simulink model "FailureModesGen"  (R2018b)
settings: configuration reference "Physics" (kept outside this file)
model workspace (MAT data in the model file):
  m = 1000
values from neighbouring files (symbols this model uses):
  P_SimDetectFailures = 1    [FailureModesGen.sldd]
  P_SimFailureBrakeMode = 0.0    [FailureModesGen.sldd]
  P_SimFailureBrakeStepEndTime_s = 200.0    [FailureModesGen.sldd]
  P_SimFailureBrakeStepTime_s = -1.0    [FailureModesGen.sldd]
  P_SimFailureIMU1Mode = 0.0    [FailureModesGen.sldd]
  P_SimFailureIMU1StepEndTime_s = 200.0    [FailureModesGen.sldd]
  P_SimFailureIMU1StepTime_s = -1.0    [FailureModesGen.sldd]
  P_SimFailureIMU2Mode = 0.0    [FailureModesGen.sldd]
  P_SimFailureIMU2StepEndTime_s = 200.0    [FailureModesGen.sldd]
  P_SimFailureIMU2StepTime_s = -1.0    [FailureModesGen.sldd]
  P_SimFailureLoc1Mode = 0.0    [FailureModesGen.sldd]
  P_SimFailureLoc1StepEndTime_s = 200.0    [FailureModesGen.sldd]
  P_SimFailureLoc1StepTime_s = -1.0    [FailureModesGen.sldd]
  P_SimFailureLoc2Mode = 0.0    [FailureModesGen.sldd]
  P_SimFailureLoc2StepEndTime_s = 200.0    [FailureModesGen.sldd]
  P_SimFailureLoc2StepTime_s = -1.0    [FailureModesGen.sldd]
  P_SimFailureModeDetectionDelay = 6.0    [FailureModesGen.sldd]
  P_SimFailureSteeringActuatorMode = 0.0    [FailureModesGen.sldd]
  P_SimFailureSteeringActuatorStepEndTime_s = 200.0    [FailureModesGen.sldd]
  P_SimFailureSteeringActuatorStepTime_s = -1.0    [FailureModesGen.sldd]
  P_SimFailureSteeringMode = 0.0    [FailureModesGen.sldd]
  P_SimFailureSteeringStepEndTime_s = 200.0    [FailureModesGen.sldd]
  P_SimFailureSteeringStepTime_s = -1.0    [FailureModesGen.sldd]
  P_SimFailureTorqueMode = 0.0    [FailureModesGen.sldd]
  P_SimFailureTorqueStepEndTime_s = 200.0    [FailureModesGen.sldd]
  P_SimFailureTorqueStepTime_s = -1.0    [FailureModesGen.sldd]
  P_SimFailureVehicleMode = 0.0    [FailureModesGen.sldd]
  P_SimFailureVehicleStepEndTime_s = 200.0    [FailureModesGen.sldd]
  P_SimFailureVehicleStepTime_s = -1.0    [FailureModesGen.sldd]
  P_SimFailureVel1Mode = 0.0    [FailureModesGen.sldd]
  P_SimFailureVel1StepEndTime_s = 200.0    [FailureModesGen.sldd]
  P_SimFailureVel1StepTime_s = -1.0    [FailureModesGen.sldd]
  P_SimFailureVel2Mode = 0.0    [FailureModesGen.sldd]
  P_SimFailureVel2StepEndTime_s = 200.0    [FailureModesGen.sldd]
  P_SimFailureVel2StepTime_s = -1.0    [FailureModesGen.sldd]
  P_SimFailureWheelspeedsMode = 0.0    [FailureModesGen.sldd]
  P_SimFailureWheelspeedsStepEndTime_s = 200.0    [FailureModesGen.sldd]
  P_SimFailureWheelspeedsStepTime_s = -1.0    [FailureModesGen.sldd]
settings Model: DataDictionary=FailureModesGen.sldd  PauseTimes=9.280  Creator=wischnewski  LastModifiedBy=ge34qer

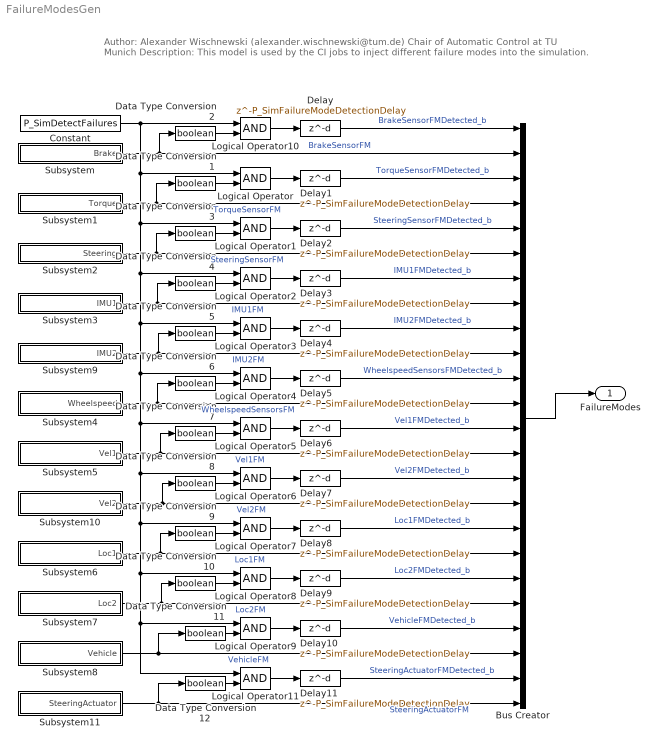
== system FailureModesGen ==
  note: Author: Alexander Wischnewski (alexander.wischnewski@tum.de)
      | Chair of Automatic Control at TU Munich
      |
      | Description: This model is used by the CI jobs to inject different failure modes into the simulation.
  Bus Creator : BusCreator  Inputs=24
  Constant : Constant  Value=P_SimDetectFailures
  Data Type Conversion{1..12} (12 alike) : DataTypeConversion  OutDataTypeStr=boolean
  Delay{,1..11} (12 alike) : Delay  DelayLength=P_SimFailureModeDetectionDelay  InitialCondition=0
  Logical Operator{,1..11} (12 alike) : Logic  AllPortsSameDT=off  OutDataTypeStr=boolean
  Subsystem : Subsystem
  Subsystem1 : Subsystem
  Subsystem10 : Subsystem
  Subsystem11 : Subsystem
  Subsystem2 : Subsystem
  Subsystem3 : Subsystem
  Subsystem4 : Subsystem
  Subsystem5 : Subsystem
  Subsystem6 : Subsystem
  Subsystem7 : Subsystem
  Subsystem8 : Subsystem
  Subsystem9 : Subsystem
  FailureModes : Outport  OutDataTypeStr=Bus: FailureModes
  wires:
  Logical Operator10/1 -> Delay/1
  Delay/1 -> Bus Creator/1  "BrakeSensorFMDetected_b"
  Subsystem/1(Brake) -> Data Type Conversion2/1, Bus Creator/2  "BrakeSensorFM"
  Subsystem1/1(Torque) -> Data Type Conversion1/1, Bus Creator/4  "TorqueSensorFM"
  Delay1/1 -> Bus Creator/3  "TorqueSensorFMDetected_b"
  Subsystem2/1(Steering) -> Data Type Conversion3/1, Bus Creator/6  "SteeringSensorFM"
  Logical Operator1/1 -> Delay2/1
  Delay2/1 -> Bus Creator/5  "SteeringSensorFMDetected_b"
  Delay3/1 -> Bus Creator/7  "IMU1FMDetected_b"
  Subsystem3/1(IMU1) -> Data Type Conversion4/1, Bus Creator/8  "IMU1FM"
  Logical Operator3/1 -> Delay4/1
  Delay4/1 -> Bus Creator/9  "IMU2FMDetected_b"
  Subsystem9/1(IMU2) -> Data Type Conversion5/1, Bus Creator/10  "IMU2FM"
  Logical Operator4/1 -> Delay5/1
  Subsystem4/1(Wheelspeed) -> Data Type Conversion6/1, Bus Creator/12  "WheelspeedSensorsFM"
  Delay5/1 -> Bus Creator/11  "WheelspeedSensorsFMDetected_b"
  Logical Operator5/1 -> Delay6/1
  Delay6/1 -> Bus Creator/13  "Vel1FMDetected_b"
  Subsystem5/1(Vel1) -> Data Type Conversion7/1, Bus Creator/14  "Vel1FM"
  Logical Operator6/1 -> Delay7/1
  Delay7/1 -> Bus Creator/15  "Vel2FMDetected_b"
  Subsystem10/1(Vel2) -> Data Type Conversion8/1, Bus Creator/16  "Vel2FM"
  Logical Operator7/1 -> Delay8/1
  Delay8/1 -> Bus Creator/17  "Loc1FMDetected_b"
  Subsystem6/1(Loc1) -> Data Type Conversion9/1, Bus Creator/18  "Loc1FM"
  Logical Operator8/1 -> Delay9/1
  Delay9/1 -> Bus Creator/19  "Loc2FMDetected_b"
  Subsystem7/1(Loc2) -> Data Type Conversion10/1, Bus Creator/20  "Loc2FM"
  Logical Operator9/1 -> Delay10/1
  Delay10/1 -> Bus Creator/21  "VehicleFMDetected_b"
  Subsystem8/1(Vehicle) -> Data Type Conversion11/1, Bus Creator/22  "VehicleFM"
  Bus Creator/1 -> FailureModes/1
  Constant/1 -> Logical Operator10/1, Logical Operator9/1, Logical Operator11/1, Logical Operator8/1, Logical Operator7/1, Logical Operator6/1, Logical Operator5/1, Logical Operator4/1, Logical Operator3/1, Logical Operator2/1, Logical Operator1/1, Logical Operator/1
  Logical Operator/1 -> Delay1/1
  Logical Operator2/1 -> Delay3/1
  Data Type Conversion1/1 -> Logical Operator/2
  Data Type Conversion2/1 -> Logical Operator10/2
  Data Type Conversion3/1 -> Logical Operator1/2
  Data Type Conversion4/1 -> Logical Operator2/2
  Data Type Conversion5/1 -> Logical Operator3/2
  Data Type Conversion6/1 -> Logical Operator4/2
  Data Type Conversion7/1 -> Logical Operator5/2
  Data Type Conversion8/1 -> Logical Operator6/2
  Data Type Conversion9/1 -> Logical Operator7/2
  Data Type Conversion10/1 -> Logical Operator8/2
  Data Type Conversion11/1 -> Logical Operator9/2
  Data Type Conversion12/1 -> Logical Operator11/2
  Subsystem11/1(SteeringActuator) -> Bus Creator/24, Data Type Conversion12/1  "SteeringActuatorFM"
  Logical Operator11/1 -> Delay11/1
  Delay11/1 -> Bus Creator/23  "SteeringActuatorFMDetected_b"

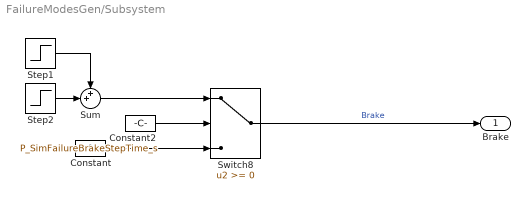
== system FailureModesGen/Subsystem ==
  Constant : Constant  Value=0
  Constant2 : Constant  Value=P_SimFailureBrakeStepTime_s
  Step1 : Step  Time=P_SimFailureBrakeStepTime_s  After=P_SimFailureBrakeMode  SampleTime=0
  Step2 : Step  Time=P_SimFailureBrakeStepEndTime_s  After=-P_SimFailureBrakeMode  SampleTime=0
  Sum : Sum  Inputs=++|
  Switch8 : Switch
  Brake : Outport
  wires:
  Constant/1 -> Switch8/3
  Sum/1 -> Switch8/1
  Constant2/1 -> Switch8/2
  Switch8/1 -> Brake/1  "Brake"
  Step1/1 -> Sum/1
  Step2/1 -> Sum/2

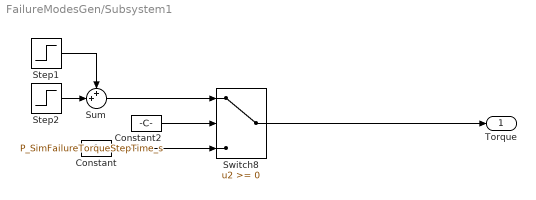
== system FailureModesGen/Subsystem1 ==
  Constant : Constant  Value=0
  Constant2 : Constant  Value=P_SimFailureTorqueStepTime_s
  Step1 : Step  Time=P_SimFailureTorqueStepTime_s  After=P_SimFailureTorqueMode  SampleTime=0
  Step2 : Step  Time=P_SimFailureTorqueStepEndTime_s  After=-P_SimFailureTorqueMode  SampleTime=0
  Sum : Sum  Inputs=++|
  Switch8 : Switch
  Torque : Outport
  wires:
  Constant/1 -> Switch8/3
  Sum/1 -> Switch8/1
  Constant2/1 -> Switch8/2
  Switch8/1 -> Torque/1
  Step2/1 -> Sum/2
  Step1/1 -> Sum/1

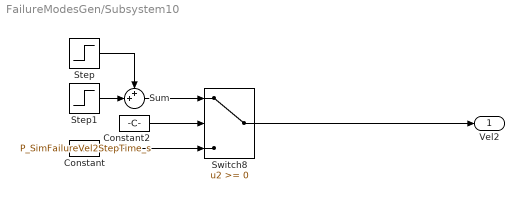
== system FailureModesGen/Subsystem10 ==
  Constant : Constant  Value=0
  Constant2 : Constant  Value=P_SimFailureVel2StepTime_s
  Step : Step  Time=P_SimFailureVel2StepTime_s  After=P_SimFailureVel2Mode  SampleTime=0
  Step1 : Step  Time=P_SimFailureVel2StepEndTime_s  After=-P_SimFailureVel2Mode  SampleTime=0
  Sum : Sum  Inputs=++|
  Switch8 : Switch
  Vel2 : Outport
  wires:
  Constant/1 -> Switch8/3
  Constant2/1 -> Switch8/2
  Switch8/1 -> Vel2/1
  Step/1 -> Sum/1
  Step1/1 -> Sum/2
  Sum/1 -> Switch8/1

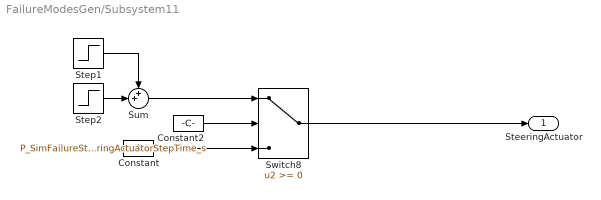
== system FailureModesGen/Subsystem11 ==
  Constant : Constant  Value=0
  Constant2 : Constant  Value=P_SimFailureSteeringActuatorStepTime_s
  Step1 : Step  Time=P_SimFailureSteeringActuatorStepTime_s  After=P_SimFailureSteeringActuatorMode  SampleTime=0
  Step2 : Step  Time=P_SimFailureSteeringActuatorStepEndTime_s  After=-P_SimFailureSteeringActuatorMode  SampleTime=0
  Sum : Sum  Inputs=++|
  Switch8 : Switch
  SteeringActuator : Outport
  wires:
  Constant/1 -> Switch8/3
  Sum/1 -> Switch8/1
  Constant2/1 -> Switch8/2
  Switch8/1 -> SteeringActuator/1
  Step2/1 -> Sum/2
  Step1/1 -> Sum/1

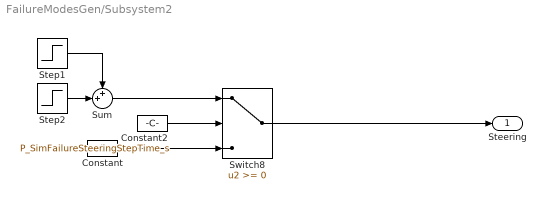
== system FailureModesGen/Subsystem2 ==
  Constant : Constant  Value=0
  Constant2 : Constant  Value=P_SimFailureSteeringStepTime_s
  Step1 : Step  Time=P_SimFailureSteeringStepTime_s  After=P_SimFailureSteeringMode  SampleTime=0
  Step2 : Step  Time=P_SimFailureSteeringStepEndTime_s  After=-P_SimFailureSteeringMode  SampleTime=0
  Sum : Sum  Inputs=++|
  Switch8 : Switch
  Steering : Outport
  wires:
  Constant/1 -> Switch8/3
  Sum/1 -> Switch8/1
  Constant2/1 -> Switch8/2
  Switch8/1 -> Steering/1
  Step2/1 -> Sum/2
  Step1/1 -> Sum/1

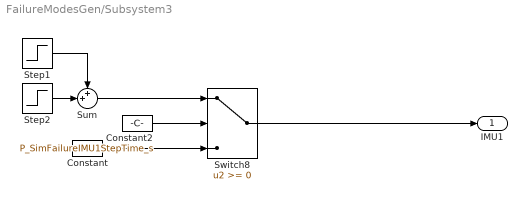
== system FailureModesGen/Subsystem3 ==
  Constant : Constant  Value=0
  Constant2 : Constant  Value=P_SimFailureIMU1StepTime_s
  Step1 : Step  Time=P_SimFailureIMU1StepTime_s  After=P_SimFailureIMU1Mode  SampleTime=0
  Step2 : Step  Time=P_SimFailureIMU1StepEndTime_s  After=-P_SimFailureIMU1Mode  SampleTime=0
  Sum : Sum  Inputs=++|
  Switch8 : Switch
  IMU1 : Outport
  wires:
  Constant/1 -> Switch8/3
  Sum/1 -> Switch8/1
  Constant2/1 -> Switch8/2
  Switch8/1 -> IMU1/1
  Step2/1 -> Sum/2
  Step1/1 -> Sum/1

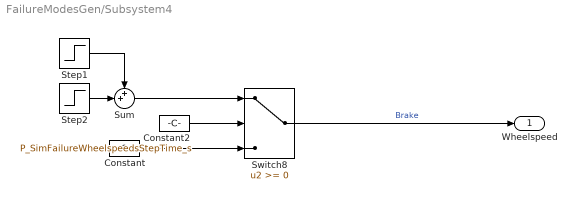
== system FailureModesGen/Subsystem4 ==
  Constant : Constant  Value=0
  Constant2 : Constant  Value=P_SimFailureWheelspeedsStepTime_s
  Step1 : Step  Time=P_SimFailureWheelspeedsStepTime_s  After=P_SimFailureWheelspeedsMode  SampleTime=0
  Step2 : Step  Time=P_SimFailureWheelspeedsStepEndTime_s  After=-P_SimFailureWheelspeedsMode  SampleTime=0
  Sum : Sum  Inputs=++|
  Switch8 : Switch
  Wheelspeed : Outport
  wires:
  Constant/1 -> Switch8/3
  Sum/1 -> Switch8/1
  Constant2/1 -> Switch8/2
  Switch8/1 -> Wheelspeed/1  "Brake"
  Step2/1 -> Sum/2
  Step1/1 -> Sum/1

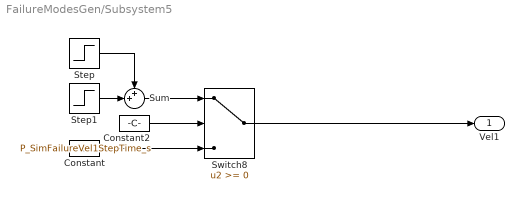
== system FailureModesGen/Subsystem5 ==
  Constant : Constant  Value=0
  Constant2 : Constant  Value=P_SimFailureVel1StepTime_s
  Step : Step  Time=P_SimFailureVel1StepTime_s  After=P_SimFailureVel1Mode  SampleTime=0
  Step1 : Step  Time=P_SimFailureVel1StepEndTime_s  After=-P_SimFailureVel1Mode  SampleTime=0
  Sum : Sum  Inputs=++|
  Switch8 : Switch
  Vel1 : Outport
  wires:
  Constant/1 -> Switch8/3
  Constant2/1 -> Switch8/2
  Switch8/1 -> Vel1/1
  Step/1 -> Sum/1
  Step1/1 -> Sum/2
  Sum/1 -> Switch8/1

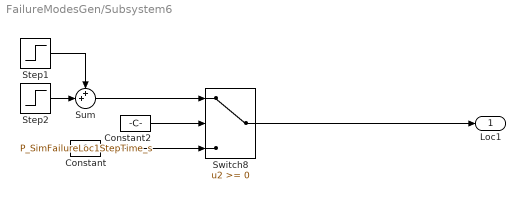
== system FailureModesGen/Subsystem6 ==
  Constant : Constant  Value=0
  Constant2 : Constant  Value=P_SimFailureLoc1StepTime_s
  Step1 : Step  Time=P_SimFailureLoc1StepTime_s  After=P_SimFailureLoc1Mode  SampleTime=0
  Step2 : Step  Time=P_SimFailureLoc1StepEndTime_s  After=-P_SimFailureLoc1Mode  SampleTime=0
  Sum : Sum  Inputs=++|
  Switch8 : Switch
  Loc1 : Outport
  wires:
  Constant/1 -> Switch8/3
  Sum/1 -> Switch8/1
  Constant2/1 -> Switch8/2
  Switch8/1 -> Loc1/1
  Step2/1 -> Sum/2
  Step1/1 -> Sum/1

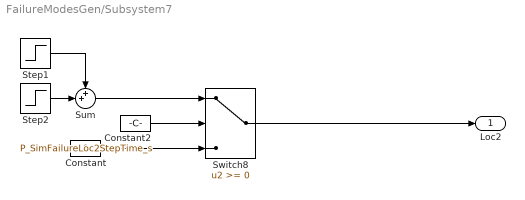
== system FailureModesGen/Subsystem7 ==
  Constant : Constant  Value=0
  Constant2 : Constant  Value=P_SimFailureLoc2StepTime_s
  Step1 : Step  Time=P_SimFailureLoc2StepTime_s  After=P_SimFailureLoc2Mode  SampleTime=0
  Step2 : Step  Time=P_SimFailureLoc2StepEndTime_s  After=-P_SimFailureLoc2Mode  SampleTime=0
  Sum : Sum  Inputs=++|
  Switch8 : Switch
  Loc2 : Outport
  wires:
  Constant/1 -> Switch8/3
  Sum/1 -> Switch8/1
  Constant2/1 -> Switch8/2
  Switch8/1 -> Loc2/1
  Step2/1 -> Sum/2
  Step1/1 -> Sum/1

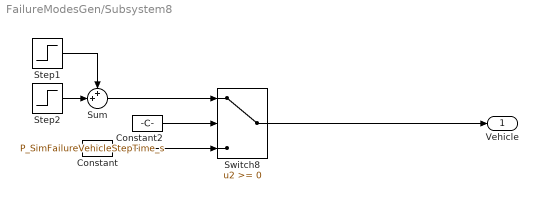
== system FailureModesGen/Subsystem8 ==
  Constant : Constant  Value=0
  Constant2 : Constant  Value=P_SimFailureVehicleStepTime_s
  Step1 : Step  Time=P_SimFailureVehicleStepTime_s  After=P_SimFailureVehicleMode  SampleTime=0
  Step2 : Step  Time=P_SimFailureVehicleStepEndTime_s  After=-P_SimFailureVehicleMode  SampleTime=0
  Sum : Sum  Inputs=++|
  Switch8 : Switch
  Vehicle : Outport
  wires:
  Constant/1 -> Switch8/3
  Sum/1 -> Switch8/1
  Constant2/1 -> Switch8/2
  Switch8/1 -> Vehicle/1
  Step2/1 -> Sum/2
  Step1/1 -> Sum/1

== system FailureModesGen/Subsystem9 ==
  Constant : Constant  Value=0
  Constant2 : Constant  Value=P_SimFailureIMU2StepTime_s
  Step1 : Step  Time=P_SimFailureIMU2StepTime_s  After=P_SimFailureIMU2Mode  SampleTime=0
  Step2 : Step  Time=P_SimFailureIMU2StepEndTime_s  After=-P_SimFailureIMU2Mode  SampleTime=0
  Sum : Sum  Inputs=++|
  Switch8 : Switch
  IMU2 : Outport
  wires:
  Constant/1 -> Switch8/3
  Sum/1 -> Switch8/1
  Constant2/1 -> Switch8/2
  Switch8/1 -> IMU2/1
  Step2/1 -> Sum/2
  Step1/1 -> Sum/1
